simulink model "Exercitiu"  (R2024b)
settings: Solver=VariableStepAuto  StartTime=0.0  StopTime=10.0  RelTol=1e-3
values from neighbouring files (symbols this model uses):
  C = 1    [Lab5.m]
  L = 1    [Lab5.m]
settings Model: Creator=rares  LastModifiedBy=rares

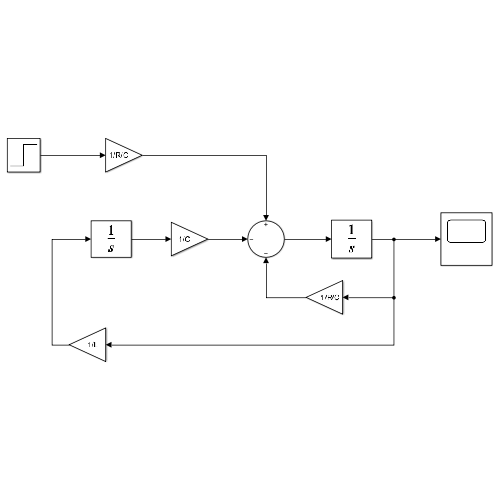
[thumbnail: Simulink's stored preview of the top-level diagram]
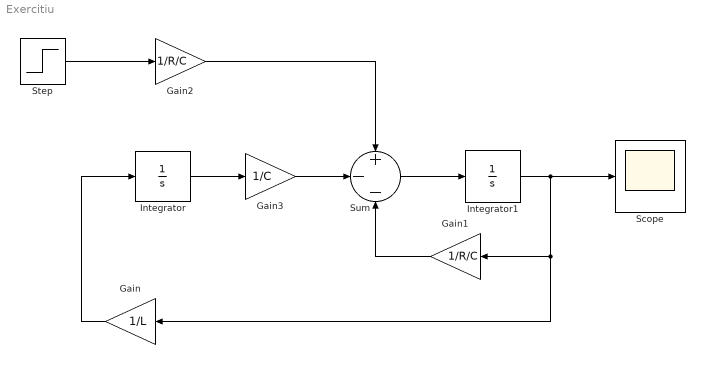
== system Exercitiu ==
  Gain : Gain  Gain=1/L
  Gain1 : Gain  Gain=1/R/C
  Gain2 : Gain  Gain=1/R/C
  Gain3 : Gain  Gain=1/C
  Integrator : Integrator
  Integrator1 : Integrator
  Scope : Scope
  Step : Step  SampleTime=0
  Sum : Sum  Inputs=+--
  wires:
  Integrator1/1 -> Scope/1, Gain/1, Gain1/1
  Gain/1 -> Integrator/1
  Sum/1 -> Integrator1/1
  Gain1/1 -> Sum/3
  Gain2/1 -> Sum/1
  Gain3/1 -> Sum/2
  Integrator/1 -> Gain3/1
  Step/1 -> Gain2/1
